simulink model "multipacketSystemDataPackager"  (R2012b)
settings: Solver=FixedStepDiscrete  StartTime=0.0  StopTime=10.0  FixedStep=0.001  RelTol=1e-3
libraries: simulink x1, xpclib x1
settings Model: BufferReuse=off  Creator=gilja  LastModifiedBy=Chethan
settings SolverCC: EnableConcurrentExecution=on  ConcurrentTasks=on
settings DataIOCC: SaveOutput=off  SignalLogging=off  SaveTime=off
settings OptimizationCC: InlineParams=on  InlineInvariantSignals=on  OptimizeBlockIOStorage=off  BufferReuse=off  ExpressionFolding=off  LocalBlockOutputs=off  SimCompilerOptimization=On
settings HardwareCC: ProdIntDivRoundTo=Zero  ProdEndianess=LittleEndian  ProdHWDeviceType=Generic->32-bit x86 compatible
settings ModelReferenceCC: ModelReferenceNumInstancesAllowed=Single  ModelReferenceMinAlgLoopOccurrences=on
settings RTWCC: SystemTargetFile=xpctarget.tlc  TemplateMakefile=xpc_default_tmf  Description=xPC Target  ProcessScript=xpctarget_make_rtw_hook  RTWCompilerOptimization=On
settings CodeAppCC: MaxIdLength=62
settings xpcTargetCC: TargetFcnLib=ansi_tfl_table_tmw.mat  CodeReplacementLibrary=XPC_BLAS  ParMdlRefBuildCompliant=on  ConcurrentExecutionCompliant=on  CombineSignalStateStructs=off  GRTInterface=on  RL32LogTETModifier=off  xPCTaskExecutionProfile=off  xPCRL32EventNumber=5000  xPCisDownloadable=off  xPCLoadParamSetFile=off  xPCConcurrentTasks=off  xPCEnableSFAnimation=off

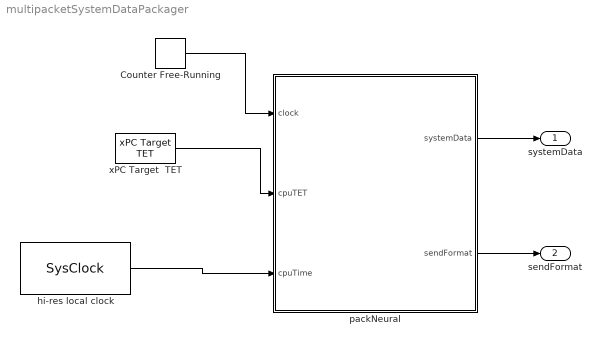
== system multipacketSystemDataPackager ==
  Counter Free-Running : simulink/Sources/Counter Free-Running  NumBits=32  tsamp=-1
  hi-res local clock : S-Function  InitFcn=try, set_param(gcb,'FunctionName','SysClock'), end  FunctionName=SysClock  SFunctionModules=SysClock_wrapper  EnableBusSupport=off  mask(S-Function Builder){}
      mask help: Simulink:masks:SFunctionBuilder_MD
      mask init:
      | val = [[.9  0.75 0.75 1 1 .9 .9 1]',[1 1 0.75 0.75 .9 .9 1 .9]'];try , sys = get_param(gcb,'SfunBuilderFcnName');if isempty(sys), sys = get_param(gcb,'FunctionName'); end,catch, sys = get_param(gcb,'FunctionName'); end
      settings: CopyFcn=set_param(gcbh,'LinkStatus','none')  PreSaveFcn=try, set_param(gcb,'FunctionName','SysClock'), end  OpenFcn=sfunctionwizard(gcbh)
      mask Display: plot(val(:,1),val(:,2)),disp(sys), port_label('output',1,'sysClk')
  packNeural : MATLAB Function  TreatAsAtomicUnit=on
  "xPC Target  TET " : xpclib/Misc./xPC Target  TET   ts=0.001
  systemData : Outport  OutDataTypeStr=Bus: fileLoggerFormatAndData  BusOutputAsStruct=on
  sendFormat : Outport  Port=2  BusOutputAsStruct=on
  wires:
  packNeural/1(systemData) -> systemData/1
  "xPC Target  TET "/1 -> packNeural/2(cpuTET)
  packNeural/2(sendFormat) -> sendFormat/1
  hi-res local clock/1 -> packNeural/3(cpuTime)
  Counter Free-Running/1 -> packNeural/1(clock)

== matlab function multipacketSystemDataPackager/packNeural ==
  data: systemData output Bus: fileLoggerFormatAndData size=1; clock input; cpuTET input; cpuTime input; sendFormat output
function [systemData, sendFormat] = packNeural(clock, cpuTET, cpuTime)
%#codegen

VERSION_ID = single(1.1);

outputstring = 'system';

%% PACK DATA FOR UDP OUTPUT
systemData = packFileLoggerFormatAndData(outputstring, ...
    'systemDataPackage', VERSION_ID, ...
    'clock', clock, ...
    'cpuTET', cpuTET, ...
    'cpuTimes', cpuTime ...
    );

systemData.data.send = true;

if mod(clock, 1000) == 0
    sendFormat = true;
else
    sendFormat = false;
end
